simulink model "hierarchical_controll"  (R2022b)
settings: Solver=ode45  StartTime=0.0  StopTime=40  RelTol=1e-3
values from neighbouring files (symbols this model uses):
  d0 = 3.5    [planner.m]
  e_3 = [0 0 1]'    [main.m]
  g = 9.81    [main.m]
  Ib = diag([1.2416 1.2416 2*1.2416])    [main.m]
  K_attr = 0.8    [planner.m]
  K_rep = 0.6    [planner.m]
  Kp = diag([100 100 100])    [main.m]
  Kr = diag([20 20 3.5])    [main.m]
  Kv = diag([8 8 8])    [main.m]
  Kw = diag([5 6.5 2.5])    [main.m]
  lin_vel_0 = [dot_x0 dot_y0 dot_z0]    [planner.m]
  mass = 1.2    [main.m]
  obstacle_points_total = obstacle_points_total'    [planner.m]
  orient_0 = [0 0 0]    [planner.m]
  pos_0 = [x0 y0 z0]    [planner.m]
  pos_fin = [xf yf zf]    [planner.m]
  Ts = 0.001    [main.m]
  uT_0 = 11.772    [main.m]
  w_bb_0 = [0 0 0]    [planner.m]
libraries: uavsimlib x3, robotcorelib x2, uavutilslib x2, eeGeneralControl x1
settings Model: Creator=fabioruggiero  LastModifiedBy=anton
settings OptimizationCC: ReuseModelBlockBuffer=on
settings ModelReferenceCC: EnableRefExpFcnMdlSchedulingChecks=on

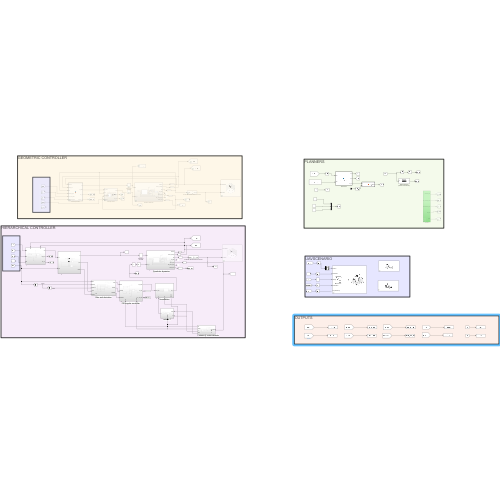
[thumbnail: Simulink's stored preview of the top-level diagram]
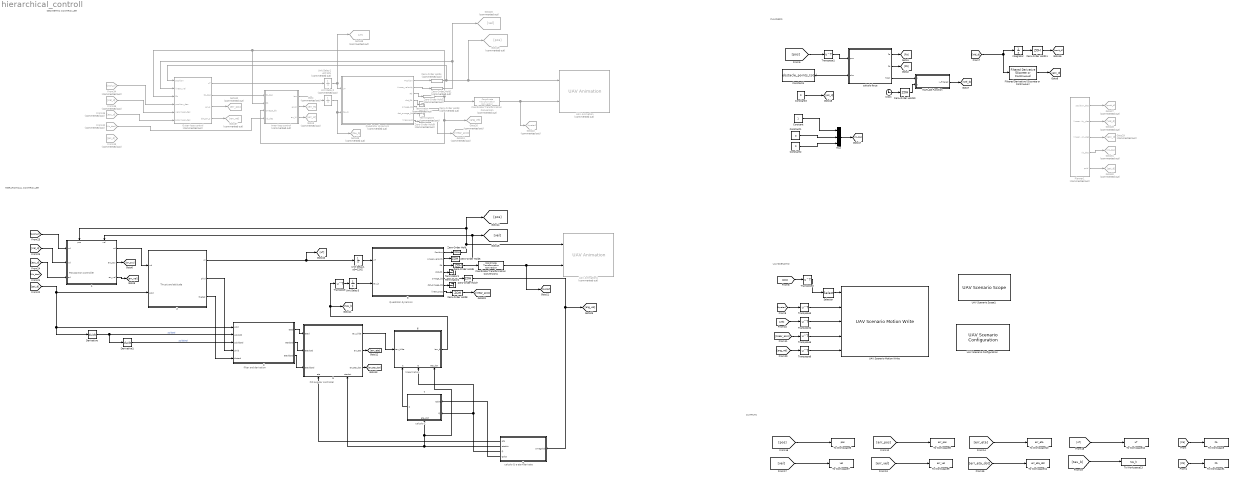
== system hierarchical_controll ==
  note: calcolo Q e eta+derivate
  note: calcolo C
  note: linearization
  note: PID angular controller
  note: Quadrotor dynamics
  note: filter and derivation
  note: Thrust and attitude
  note: PID position controller
  note: PLANNERS
  note: HIERARCHICAL CONTROLLER
  note: GEOMETRIC CONTROLLER
  note: UAVSCENARIO
  note: OUTPUTS
  "1                                                               " : Subsystem
      settings: PortSchema="{\"entries\":[{\"content\":{\"sides\":[{\"content\":{\"connectorIds\":[\"In1\",\"In2\",\"In3\"]},\"type\":\"ConnectorPlacement.EquallySpacedRectSide\",\"uuid\":\"85e0d77d-a667-4893-9520-464dcfab6198\"},{\"content\":{\"connectorIds\":[\"Out1\",\"Out2\",\"Out3\"],\"side\":\"RIGHT\"},\"type\":\"ConnectorPlacement.EquallySpacedRectSide\",\"uuid\":\"778112c6-e857-467f-a494-37829ee7f6de\"},{\"content\":{\"connectorIds\":[\"In4\",\"In5\"],\"side\":\"TOP\"},\"type\":\"ConnectorPlacement.EquallySpacedRectSide\",\"uuid\":\"7a58fbc8-384a-41ea-ad35-507457b1f60b\"}]},\"type\":\"ConnectorPlacement.EquallySpacedConnector\",\"uuid\":\"a6f9beb4-828c-454c-887a-520afea17d8a\"}],\"packageUris\":[\"http://schema.mathworks.com/mf0/Connector/R2020b\"],\"version\":\"1.0\"}"
  "2                                                       " : Subsystem
  "3                                                                                " : Subsystem
  "4                                                                          " : Subsystem
  "5                                                                   " : Subsystem
      settings: PortSchema="{\"entries\":[{\"content\":{\"sides\":[{\"content\":{\"connectorIds\":[\"In1\",\"In2\",\"In3\"]},\"type\":\"ConnectorPlacement.EquallySpacedRectSide\",\"uuid\":\"65edaed1-88f7-4380-a3c2-d91c382e58d8\"},{\"content\":{\"connectorIds\":[\"Out1\",\"Out2\",\"Out3\"],\"side\":\"RIGHT\"},\"type\":\"ConnectorPlacement.EquallySpacedRectSide\",\"uuid\":\"b4927c3a-556e-4efb-b7a2-196eb11d91c2\"},{\"content\":{\"connectorIds\":[],\"side\":\"TOP\"},\"type\":\"ConnectorPlacement.EquallySpacedRectSide\",\"uuid\":\"d0d93e72-ef33-404e-bf49-2a921e5b1f46\"},{\"content\":{\"connectorIds\":[\"In4\",\"In5\"],\"side\":\"BOTTOM\"},\"type\":\"ConnectorPlacement.EquallySpacedRectSide\",\"uuid\":\"fc2b4b79-e5bc-46f9-b483-cd3a784daa2c\"}]},\"type\":\"ConnectorPlacement.EquallySpacedConnector\",\"uuid\":\"3b418c0f-1ef1-41d2-9d0b-065cc025c1dc\"}],\"packageUris\":[\"http://schema.mathworks.com/mf0/Connector/R2020b\"],\"version\":\"1.0\"}"
  "6                                                          " : Subsystem
      settings: PortSchema="{\"entries\":[{\"content\":{\"sides\":[{\"content\":{\"connectorIds\":[\"In1\"]},\"type\":\"ConnectorPlacement.EquallySpacedRectSide\",\"uuid\":\"0beb0235-60e3-41f7-812a-43c156a669e6\"},{\"content\":{\"connectorIds\":[\"Out1\"],\"side\":\"RIGHT\"},\"type\":\"ConnectorPlacement.EquallySpacedRectSide\",\"uuid\":\"de9ad457-04ca-4167-913f-fe2cc1e03613\"},{\"content\":{\"connectorIds\":[],\"side\":\"TOP\"},\"type\":\"ConnectorPlacement.EquallySpacedRectSide\",\"uuid\":\"f1328202-7222-41d3-b6d6-2d5d11bea743\"},{\"content\":{\"connectorIds\":[\"In2\",\"In3\",\"In4\"],\"side\":\"BOTTOM\"},\"type\":\"ConnectorPlacement.EquallySpacedRectSide\",\"uuid\":\"eb41c250-0583-48fd-9f70-967dbb920771\"}]},\"type\":\"ConnectorPlacement.EquallySpacedConnector\",\"uuid\":\"65996137-7811-4a08-986c-c256136c93e4\"}],\"packageUris\":[\"http://schema.mathworks.com/mf0/Connector/R2020b\"],\"version\":\"1.0\"}"
  "7                                     " : Subsystem
      settings: PortSchema="{\"entries\":[{\"content\":{\"sides\":[{\"content\":{\"connectorIds\":[\"In1\",\"In2\"]},\"type\":\"ConnectorPlacement.EquallySpacedRectSide\",\"uuid\":\"32eaabac-cb83-4fe8-9235-f1617512dfe4\"},{\"content\":{\"connectorIds\":[\"Out1\"],\"side\":\"RIGHT\"},\"type\":\"ConnectorPlacement.EquallySpacedRectSide\",\"uuid\":\"6410da22-b624-4417-a1de-532b1b31b04c\"},{\"content\":{\"connectorIds\":[],\"side\":\"TOP\"},\"type\":\"ConnectorPlacement.EquallySpacedRectSide\",\"uuid\":\"ac47dc5b-e2fb-44dd-8524-01f66e23453c\"},{\"content\":{\"connectorIds\":[\"In3\"],\"side\":\"BOTTOM\"},\"type\":\"ConnectorPlacement.EquallySpacedRectSide\",\"uuid\":\"bde9f19c-50b2-41fa-8bff-f203ec6c7c10\"}]},\"type\":\"ConnectorPlacement.EquallySpacedConnector\",\"uuid\":\"1596106e-62b1-4910-94cd-14b1fe3e52a0\"}],\"packageUris\":[\"http://schema.mathworks.com/mf0/Connector/R2020b\"],\"version\":\"1.0\"}"
  "8                                                            " : Subsystem
  Clock : Clock
  Constant : Constant
  Constant1 : Constant  Value=0
  Constant2 : Constant  Value=0
  Constant3 : Constant  Value=0
  Constant4 : Constant  Value=obstacle_points_total
  Coordinate Transformation Conversion : robotcorelib/Coordinate Transformation Conversion  Commented=on  InputRepresentation=Rotation Matrix  InputEulerSequence=ZYX  ShowTrVecInputPort=on  OutputRepresentation=Quaternion  OutputEulerSequence=ZYX  ShowTrVecOutputPort=on  SimulateUsing=Interpreted execution
  Coordinate Transformation Conversion1 : robotcorelib/Coordinate Transformation Conversion  InputRepresentation=Rotation Matrix  InputEulerSequence=ZYX  ShowTrVecInputPort=on  OutputRepresentation=Quaternion  OutputEulerSequence=ZYX  ShowTrVecOutputPort=on  SimulateUsing=Interpreted execution
  Derivative : Derivative
  Derivative1 : Derivative
  Filtered Derivative (Discrete or Continuous) : eeGeneralControl/Filtered Derivative (Discrete or Continuous)  K=1  T=Ts  B=inf  A=-inf  minRatio=10  init_option=Specify as parameter  x0=[0,0,0]  Ts=-1
      settings: LibrarySourceBlock=|
      | ee_sl_lib/General Control/Filtered Derivative
      | (Discrete or Continuous)
  From32 : From  Commented=on  GotoTag=xb_des
  From33 : From  Commented=on  GotoTag=psi_d
  From34 : From  Commented=on  GotoTag=posit_d
  From35 : From  Commented=on  GotoTag=acc_d
  From36 : From  Commented=on  GotoTag=Vel_d
  Goto : Goto  Commented=on  GotoTag=err_R
  Goto19 : Goto  Commented=on  GotoTag=pos
  Goto20 : Goto  Commented=on  GotoTag=vel
  Goto22 : Goto  Commented=on  GotoTag=quater
  Goto24 : Goto  Commented=on  GotoTag=linear_accc
  Goto26 : Goto  Commented=on  GotoTag=ang_vel
  Goto27 : Goto  Commented=on  GotoTag=posit_d
  Goto28 : Goto  Commented=on  GotoTag=Vel_d
  Goto29 : Goto  Commented=on  GotoTag=acc_d
  Goto3 : Goto  Commented=on  GotoTag=err_W
  Goto30 : Goto  Commented=on  GotoTag=psi_d
  Goto31 : Goto  Commented=on  GotoTag=xb_des
  Goto32 : Goto  Commented=on  GotoTag=err_pos
  Goto37 : Goto  Commented=on  GotoTag=err_vel
  Goto38 : Goto  Commented=on  GotoTag=uT
  Goto39 : Goto  Commented=on  GotoTag=tau_b
  Inner-loop control : Subsystem  Commented=on
  Integrator : Integrator  InitialCondition=pos_0
  MATLAB Function : MATLAB Function  TreatAsAtomicUnit=on
  Mux : Mux  Inputs=3
  Outer-loop control : MATLAB Function  Commented=on  TreatAsAtomicUnit=on
  Planner1 : Subsystem  Commented=on
  Quadrotor dynamics : Subsystem  Commented=on
  Selector : Selector  InputPortWidth=3  IndexOptions=Index vector (dialog)  Indices=[2 1 3]  OutputSizes=1
  Terminator : Terminator  Commented=on
  Terminator1 : Terminator
  Terminator2 : Terminator
  Terminator3 : Terminator  Commented=on
  To Workspace : ToWorkspace  VariableName=Fa  SaveFormat=Timeseries  SampleTime=-1
  To Workspace1 : ToWorkspace  VariableName=Fb  SaveFormat=Timeseries  SampleTime=-1
  To Workspace10 : ToWorkspace  VariableName=err_eta  SaveFormat=Timeseries  SampleTime=-1
  To Workspace11 : ToWorkspace  VariableName=err_eta_dot  SaveFormat=Timeseries  SampleTime=-1
  To Workspace12 : ToWorkspace  VariableName=uT  SaveFormat=Timeseries  SampleTime=-1
  To Workspace13 : ToWorkspace  VariableName=tau_b  SaveFormat=Timeseries  SampleTime=-1
  To Workspace6 : ToWorkspace  VariableName=pos  SaveFormat=Timeseries  SampleTime=-1
  To Workspace7 : ToWorkspace  VariableName=vel  SaveFormat=Timeseries  SampleTime=-1
  To Workspace8 : ToWorkspace  VariableName=err_pos  SaveFormat=Timeseries  SampleTime=-1
  To Workspace9 : ToWorkspace  VariableName=err_vel  SaveFormat=Timeseries  SampleTime=-1
  Transpose{,1..6} (7 alike) : Math  Operator=transpose
  UAV Animation : uavutilslib/UAV Animation  Commented=on  UAVType=Multirotor  UAVSize=1  InertialZDirection=Down  SampleTime=0.1
  UAV Animation1 : uavutilslib/UAV Animation  Commented=on  UAVType=Multirotor  UAVSize=2  InertialZDirection=Down  SampleTime=0.1
  UAV Scenario Configuration : uavsimlib/UAV Scenario Configuration  Priority=-1  UAVScenarioObject=piazza  SampleTime=Ts  UpdateParam=false  SensorMotionBusName='SensorMotionBus'  PlatformMotionBusName='PlatformMotionBus'  ScenarioMotionBusName='ScenarioMotionBus'  ScenarioMotionSignalName='ScenarioMotions'
  UAV Scenario Motion Write : uavsimlib/UAV Scenario Motion Write  Priority=0  PlatName='UAV_platform'  ReferenceFrame=NED
  UAV Scenario Scope1 : uavsimlib/UAV Scenario Scope  Priority=1  SensorNameTable={}  SampleTime=0.1
  Unit Delay1 u0=12N : UnitDelay  Commented=on  InitialCondition=uT_0  SampleTime=Ts
  Unit Delay1 u0=12N2 : UnitDelay  InitialCondition=uT_0  SampleTime=Ts
  Unit Delay2 : UnitDelay  Commented=on  InitialCondition=[0 0 0]  SampleTime=Ts
  Unit Delay3 : UnitDelay  InitialCondition=[0 0 0]  SampleTime=Ts
  Zero-Order Hold{,5..8,10..11} (7 alike) : ZeroOrderHold  SampleTime=Ts
  Zero-Order Hold{1..4,9} (5 alike) : ZeroOrderHold  Commented=on  SampleTime=Ts
  calcolo forza : MATLAB Function  TreatAsAtomicUnit=on
  wires:
  Outer-loop control/1(uT) -> Unit Delay1 u0=12N/1
  Unit Delay1 u0=12N/1 -> Goto38/1, Quadrotor dynamics/1(uT)
  Quadrotor dynamics/1(Position) -> Zero-Order Hold4/1
  Quadrotor dynamics/2(Linear_velocity) -> Zero-Order Hold1/1
  Quadrotor dynamics/5(omega_bb) -> Zero-Order Hold3/1
  Zero-Order Hold4/1 -> Goto19/1, UAV Animation/1, Outer-loop control/1(position)
  Zero-Order Hold1/1 -> Goto20/1, Outer-loop control/2(linear_vel)
  Quadrotor dynamics/3(Rb) -> Zero-Order Hold2/1
  Unit Delay2/1 -> Goto39/1, Quadrotor dynamics/2(tau_b)
  Quadrotor dynamics/4(dot_Rb) -> Terminator/1
  Outer-loop control/3(err_p) -> Goto32/1
  Outer-loop control/4(dot_err_p) -> Goto37/1
  Quadrotor dynamics/6(dot_omega_bb) -> Terminator3/1
  Coordinate Transformation Conversion/1 -> Goto22/1, UAV Animation/2
  Outer-loop control/2(zb_des) -> Inner-loop control/1(zb_des)
  Zero-Order Hold3/1 -> Inner-loop control/3(omega_bb), Goto26/1
  Inner-loop control/1(tau) -> Unit Delay2/1
  Inner-loop control/2(err_R) -> Goto/1
  Inner-loop control/3(err_W) -> Goto3/1
  Coordinate Transformation Conversion1/1 -> [quater], UAV Animation1/2
  "3                                                                                "/6(dot_omega_bb) -> Terminator2/1
  "3                                                                                "/4(dot_Rb) -> Terminator1/1
  "6                                                          "/1(tau_b) -> Transpose/1, [tau_b]
  Zero-Order Hold/1 -> [pos], "1                                                               "/4(pos), UAV Animation1/1
  "3                                                                                "/5(omega_bb) -> Zero-Order Hold7/1
  "3                                                                                "/3(Rb) -> Zero-Order Hold6/1
  "3                                                                                "/2(Linear_velocity) -> Zero-Order Hold5/1
  "3                                                                                "/1(Position) -> Zero-Order Hold/1
  "2                                                       "/1(ut) -> [uT], Unit Delay1 u0=12N2/1
  Zero-Order Hold5/1 -> "1                                                               "/5(vel), [vel]
  "1                                                               "/1(ud) -> "2                                                       "/1(ud)
  Derivative/1 -> Derivative1/1, "4                                                                          "/2(psidotd)  "psidotd"
  Derivative1/1 -> "4                                                                          "/3(psiddotd)  "psiddotd"
  "2                                                       "/3(thetad) -> "4                                                                          "/5(thetad)
  "2                                                       "/2(phid) -> "4                                                                          "/4(phid)
  "4                                                                          "/1(etad) -> "5                                                                   "/1(etad)
  "4                                                                          "/2(etadotd) -> "5                                                                   "/2(etadotd)
  "4                                                                          "/3(etaddotd) -> "5                                                                   "/3(etaddotd)
  "8                                                            "/1(eta) -> "5                                                                   "/4(eta)
  "8                                                            "/2(etadot) -> "5                                                                   "/5(etadot), "6                                                          "/4(eta_dot), "7                                     "/3(eta_dot)
  "5                                                                   "/1(tau_tilde) -> "6                                                          "/1(tau_tilde)
  "8                                                            "/3(Q) -> "6                                                          "/3(Q), "7                                     "/2(Q)
  "8                                                            "/4(Qdot) -> "7                                     "/1(Qdot)
  "7                                     "/1(C) -> "6                                                          "/2(C)
  Zero-Order Hold7/1 -> "8                                                            "/1(omegabb), [ang_vel]
  Unit Delay3/1 -> "3                                                                                "/2(tau_b)
  Unit Delay1 u0=12N2/1 -> "3                                                                                "/1(uT)
  [pos] -> To Workspace6/1
  [vel] -> To Workspace7/1
  [err_pos] -> To Workspace8/1
  [err_vel] -> To Workspace9/1
  [err_eta] -> To Workspace10/1
  [err_eta_dot] -> To Workspace11/1
  [uT] -> To Workspace12/1
  [tau_b] -> To Workspace13/1
  "1                                                               "/2(err_pos) -> [err_pos]
  "1                                                               "/3(err_vel) -> [err_vel]
  "5                                                                   "/2(err_eta) -> [err_eta]
  "5                                                                   "/3(err_eta_dot) -> [err_eta_dot]
  Transpose/1 -> Unit Delay3/1
  Constant4/1 -> calcolo forza/2(obs)
  [pos] -> Transpose1/1
  Transpose1/1 -> calcolo forza/1(pos)
  calcolo forza/1(Fa) -> [Fa]
  calcolo forza/2(Fb) -> [Fb]
  [Vel_d] -> Integrator/1, Filtered Derivative (Discrete or Continuous)/1
  Filtered Derivative (Discrete or Continuous)/1 -> [acc_d]
  Constant1/1 -> Mux/2
  Constant2/1 -> Mux/3
  Constant/1 -> Mux/1
  Mux/1 -> [xb_des]
  Constant3/1 -> [psi_d]
  Transpose2/1 -> Selector/1
  [pos] -> Transpose2/1
  [quater] -> Transpose3/1
  [vel] -> Transpose4/1
  Transpose4/1 -> UAV Scenario Motion Write/3
  "3                                                                                "/7(linear_accc) -> Zero-Order Hold8/1
  Quadrotor dynamics/7(linear_acc) -> Zero-Order Hold9/1
  [linear_accc] -> Transpose5/1
  Transpose5/1 -> UAV Scenario Motion Write/4
  [ang_vel] -> Transpose6/1
  Transpose6/1 -> UAV Scenario Motion Write/5
  Zero-Order Hold6/1 -> Coordinate Transformation Conversion1/1
  Transpose3/1 -> UAV Scenario Motion Write/2
  [posit_d] -> "1                                                               "/1(xd)
  [acc_d] -> "1                                                               "/3(ad)
  [Vel_d] -> "1                                                               "/2(vd)
  [psi_d] -> "2                                                       "/2(psid), "4                                                                          "/1(psid), Derivative/1
  Zero-Order Hold8/1 -> [linear_accc]
  From34/1 -> Outer-loop control/4(position_des)
  From36/1 -> Outer-loop control/5(vel_linear_des)
  From35/1 -> Outer-loop control/6(acc_linear_des)
  From32/1 -> Inner-loop control/4(xb_des)
  Zero-Order Hold9/1 -> Goto24/1
  Zero-Order Hold2/1 -> Coordinate Transformation Conversion/1, Inner-loop control/2(Rb), Outer-loop control/3(Rb)
  Clock/1 -> Zero-Order Hold10/1
  calcolo forza/3(F_tot) -> MATLAB Function/1(x)
  MATLAB Function/1(x_filtered) -> [Vel_d]
  Zero-Order Hold10/1 -> MATLAB Function/2(t)
  Zero-Order Hold11/1 -> [posit_d]
  Integrator/1 -> Zero-Order Hold11/1
  Planner1/5(psid) -> Goto30/1
  Planner1/4(xb_des) -> Goto31/1
  Planner1/3(linear_acceleration_des) -> Goto29/1
  Planner1/2(linear_velocity_des) -> Goto28/1
  Planner1/1(position_des) -> Goto27/1
  Selector/1 -> UAV Scenario Motion Write/1
  [Fa] -> To Workspace/1
  [Fb] -> To Workspace1/1

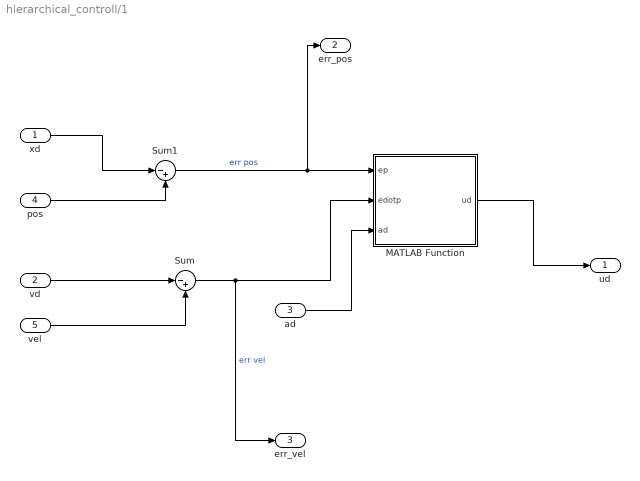
== system hierarchical_controll/1                                                                ==
  xd : Inport
  vd : Inport  Port=2
  ad : Inport  Port=3
  pos : Inport  Port=4
  vel : Inport  Port=5
  MATLAB Function : MATLAB Function  TreatAsAtomicUnit=on
  Sum : Sum  Inputs=|-+
  Sum1 : Sum  Inputs=|-+
  ud : Outport
  err_pos : Outport  Port=2
  err_vel : Outport  Port=3
  wires:
  vd/1 -> Sum/1
  vel/1 -> Sum/2
  xd/1 -> Sum1/1
  pos/1 -> Sum1/2
  Sum1/1 -> err_pos/1, MATLAB Function/1(ep)  "err pos"
  Sum/1 -> err_vel/1, MATLAB Function/2(edotp)  "err vel"
  ad/1 -> MATLAB Function/3(ad)
  MATLAB Function/1(ud) -> ud/1

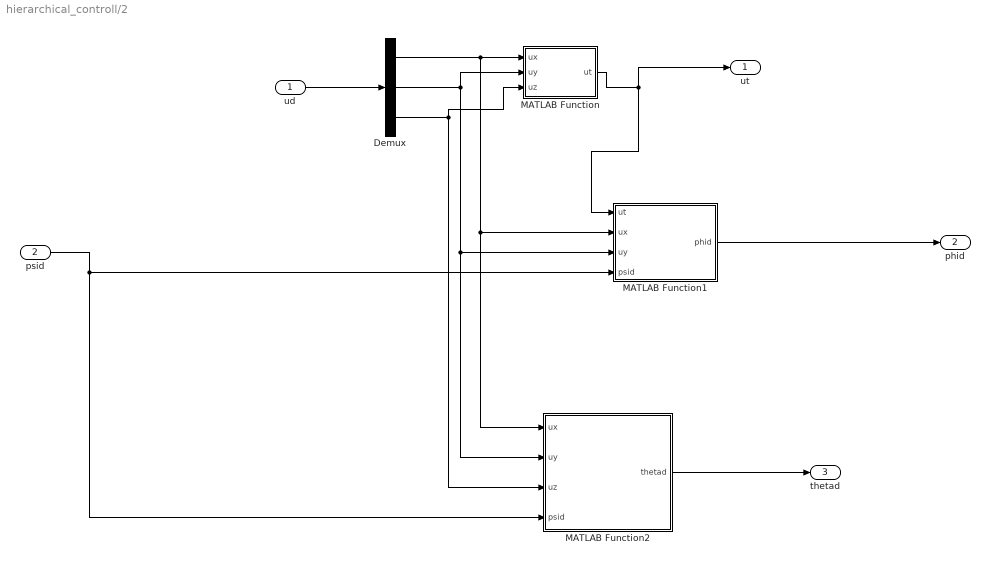
== system hierarchical_controll/2                                                        ==
  ud : Inport
  psid : Inport  Port=2
  Demux : Demux  Outputs=3
  MATLAB Function : MATLAB Function  TreatAsAtomicUnit=on
  MATLAB Function1 : MATLAB Function  TreatAsAtomicUnit=on
  MATLAB Function2 : MATLAB Function  TreatAsAtomicUnit=on
  ut : Outport
  phid : Outport  Port=2
  thetad : Outport  Port=3
  wires:
  ud/1 -> Demux/1
  Demux/1 -> MATLAB Function2/1(ux), MATLAB Function1/2(ux), MATLAB Function/1(ux)
  Demux/2 -> MATLAB Function2/2(uy), MATLAB Function1/3(uy), MATLAB Function/2(uy)
  Demux/3 -> MATLAB Function2/3(uz), MATLAB Function/3(uz)
  MATLAB Function/1(ut) -> MATLAB Function1/1(ut), ut/1
  psid/1 -> MATLAB Function2/4(psid), MATLAB Function1/4(psid)
  MATLAB Function2/1(thetad) -> thetad/1
  MATLAB Function1/1(phid) -> phid/1

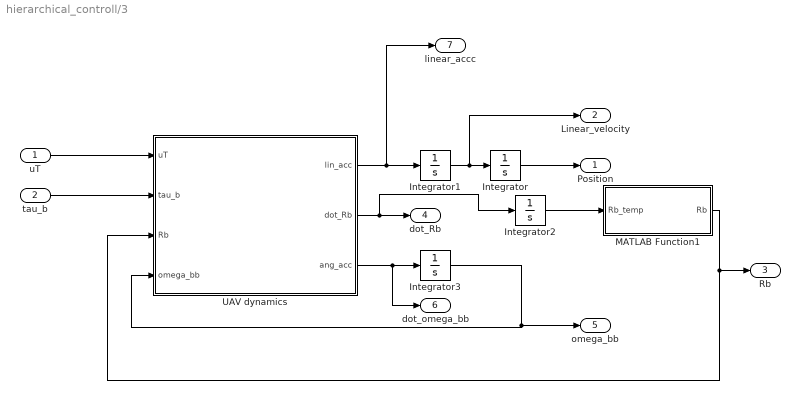
== system hierarchical_controll/3                                                                                 ==
  uT : Inport
  tau_b : Inport  Port=2
  Integrator : Integrator  InitialCondition=pos_0
  Integrator1 : Integrator  InitialCondition=lin_vel_0
  Integrator2 : Integrator  InitialCondition=eul2rotm(orient_0)
  Integrator3 : Integrator  InitialCondition=w_bb_0
  MATLAB Function1 : MATLAB Function  TreatAsAtomicUnit=on
  UAV dynamics : MATLAB Function  TreatAsAtomicUnit=on
  Position : Outport
  Linear_velocity : Outport  Port=2
  Rb : Outport  Port=3
  dot_Rb : Outport  Port=4
  omega_bb : Outport  Port=5
  dot_omega_bb : Outport  Port=6
  linear_accc : Outport  Port=7
  wires:
  Integrator2/1 -> MATLAB Function1/1(Rb_temp)
  MATLAB Function1/1(Rb) -> UAV dynamics/3(Rb), Rb/1
  UAV dynamics/2(dot_Rb) -> dot_Rb/1, Integrator2/1
  Integrator3/1 -> omega_bb/1, UAV dynamics/4(omega_bb)
  Integrator1/1 -> Integrator/1, Linear_velocity/1
  uT/1 -> UAV dynamics/1(uT)
  UAV dynamics/1(lin_acc) -> linear_accc/1, Integrator1/1
  UAV dynamics/3(ang_acc) -> Integrator3/1, dot_omega_bb/1
  Integrator/1 -> Position/1
  tau_b/1 -> UAV dynamics/2(tau_b)

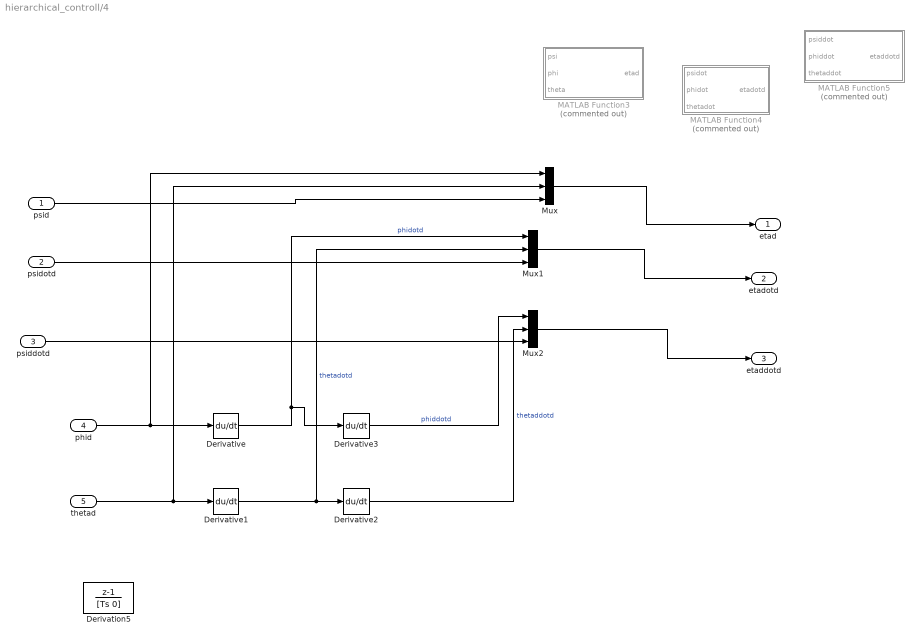
== system hierarchical_controll/4                                                                           ==
  psid : Inport
  psidotd : Inport  Port=2
  psiddotd : Inport  Port=3
  phid : Inport  Port=4
  thetad : Inport  Port=5
  Derivation5 : DiscreteTransferFcn  Numerator=[1 -1]  Denominator=[Ts 0]  SampleTime=Ts
  Derivative{,1..3} (4 alike) : Derivative
  MATLAB Function3 : MATLAB Function  Commented=on  TreatAsAtomicUnit=on
  MATLAB Function4 : MATLAB Function  Commented=on  TreatAsAtomicUnit=on
  MATLAB Function5 : MATLAB Function  Commented=on  TreatAsAtomicUnit=on
  Mux : Mux  Inputs=3
  Mux1 : Mux  Inputs=3
  Mux2 : Mux  Inputs=3
  etad : Outport
  etadotd : Outport  Port=2
  etaddotd : Outport  Port=3
  wires:
  phid/1 -> Mux/1, Derivative/1
  thetad/1 -> Mux/2, Derivative1/1
  Derivative1/1 -> Mux1/2, Derivative2/1  "thetadotd"
  Derivative/1 -> Mux1/1, Derivative3/1  "phidotd"
  Derivative3/1 -> Mux2/1  "phiddotd"
  Derivative2/1 -> Mux2/2  "thetaddotd"
  psidotd/1 -> Mux1/3
  psiddotd/1 -> Mux2/3
  Mux/1 -> etad/1
  Mux2/1 -> etaddotd/1
  psid/1 -> Mux/3
  Mux1/1 -> etadotd/1

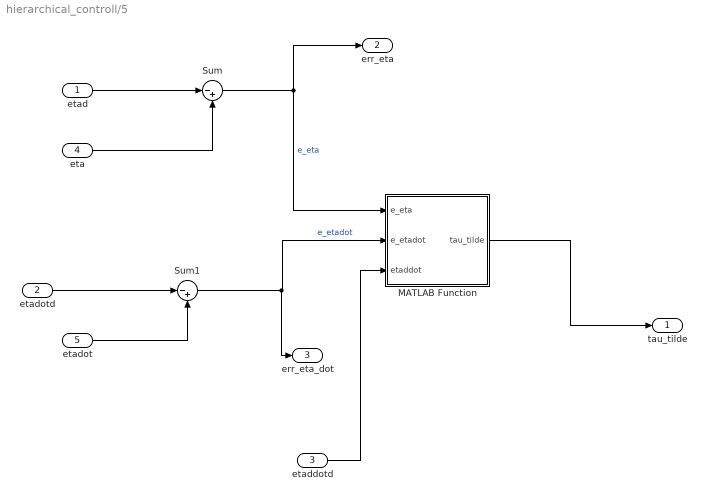
== system hierarchical_controll/5                                                                    ==
  etad : Inport
  etadotd : Inport  Port=2
  etaddotd : Inport  Port=3
  eta : Inport  Port=4
  etadot : Inport  Port=5
  MATLAB Function : MATLAB Function  TreatAsAtomicUnit=on
  Sum : Sum  Inputs=|-+
  Sum1 : Sum  Inputs=|-+
  tau_tilde : Outport
  err_eta : Outport  Port=2
  err_eta_dot : Outport  Port=3
  wires:
  etad/1 -> Sum/1
  eta/1 -> Sum/2
  etadotd/1 -> Sum1/1
  Sum/1 -> MATLAB Function/1(e_eta), err_eta/1  "e_eta"
  Sum1/1 -> err_eta_dot/1, MATLAB Function/2(e_etadot)  "e_etadot"
  MATLAB Function/1(tau_tilde) -> tau_tilde/1
  etadot/1 -> Sum1/2
  etaddotd/1 -> MATLAB Function/3(etaddot)

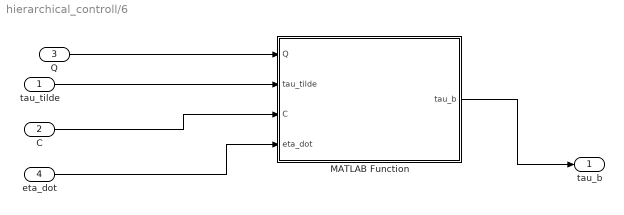
== system hierarchical_controll/6                                                           ==
  tau_tilde : Inport
  C : Inport  Port=2
  Q : Inport  Port=3
  eta_dot : Inport  Port=4
  MATLAB Function : MATLAB Function  TreatAsAtomicUnit=on
  tau_b : Outport
  wires:
  eta_dot/1 -> MATLAB Function/4(eta_dot)
  C/1 -> MATLAB Function/3(C)
  tau_tilde/1 -> MATLAB Function/2(tau_tilde)
  Q/1 -> MATLAB Function/1(Q)
  MATLAB Function/1(tau_b) -> tau_b/1

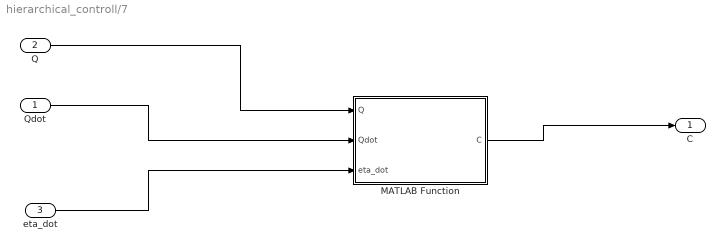
== system hierarchical_controll/7                                      ==
  Qdot : Inport
  Q : Inport  Port=2
  eta_dot : Inport  Port=3
  MATLAB Function : MATLAB Function  TreatAsAtomicUnit=on
  C : Outport
  wires:
  MATLAB Function/1(C) -> C/1
  Q/1 -> MATLAB Function/1(Q)
  Qdot/1 -> MATLAB Function/2(Qdot)
  eta_dot/1 -> MATLAB Function/3(eta_dot)

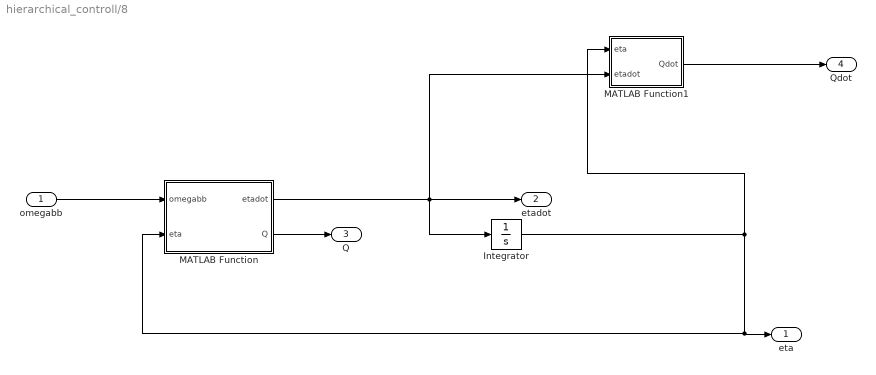
== system hierarchical_controll/8                                                             ==
  omegabb : Inport
  Integrator : Integrator  InitialCondition=[0, 0, 0]'
  MATLAB Function : MATLAB Function  TreatAsAtomicUnit=on
  MATLAB Function1 : MATLAB Function  TreatAsAtomicUnit=on
  eta : Outport
  etadot : Outport  Port=2
  Q : Outport  Port=3
  Qdot : Outport  Port=4
  wires:
  omegabb/1 -> MATLAB Function/1(omegabb)
  MATLAB Function/1(etadot) -> MATLAB Function1/2(etadot), Integrator/1, etadot/1
  MATLAB Function/2(Q) -> Q/1
  MATLAB Function1/1(Qdot) -> Qdot/1
  Integrator/1 -> MATLAB Function/2(eta), eta/1, MATLAB Function1/1(eta)

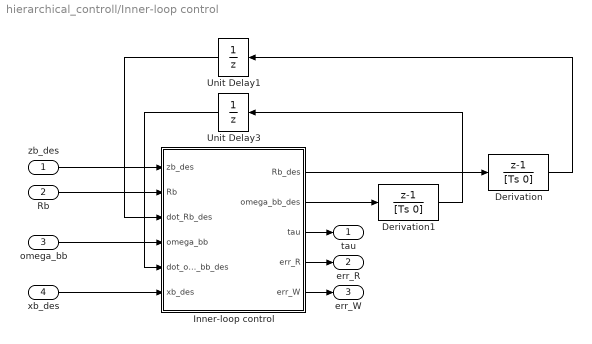
== system hierarchical_controll/Inner-loop control ==
  zb_des : Inport
  Rb : Inport  Port=2
  omega_bb : Inport  Port=3
  xb_des : Inport  Port=4
  Derivation : DiscreteTransferFcn  Numerator=[1 -1]  Denominator=[Ts 0]  InitialStates=[1 0 0;0 1 0;0 0 1]  SampleTime=Ts
  Derivation1 : DiscreteTransferFcn  Numerator=[1 -1]  Denominator=[Ts 0]  InitialStates=[0 0 0]  SampleTime=Ts
  Inner-loop control : MATLAB Function  TreatAsAtomicUnit=on
  Unit Delay1 : UnitDelay  InitialCondition=eye(3)  SampleTime=Ts
  Unit Delay3 : UnitDelay  InitialCondition=[0 0 0]  SampleTime=Ts
  tau : Outport
  err_R : Outport  Port=2
  err_W : Outport  Port=3
  wires:
  xb_des/1 -> Inner-loop control/6(xb_des)
  Inner-loop control/4(err_R) -> err_R/1
  Rb/1 -> Inner-loop control/2(Rb)
  Inner-loop control/3(tau) -> tau/1
  Unit Delay1/1 -> Inner-loop control/3(dot_Rb_des)
  Derivation1/1 -> Unit Delay3/1
  Inner-loop control/5(err_W) -> err_W/1
  Unit Delay3/1 -> Inner-loop control/5(dot_omega_bb_des)
  Derivation/1 -> Unit Delay1/1
  zb_des/1 -> Inner-loop control/1(zb_des)
  omega_bb/1 -> Inner-loop control/4(omega_bb)
  Inner-loop control/1(Rb_des) -> Derivation/1
  Inner-loop control/2(omega_bb_des) -> Derivation1/1

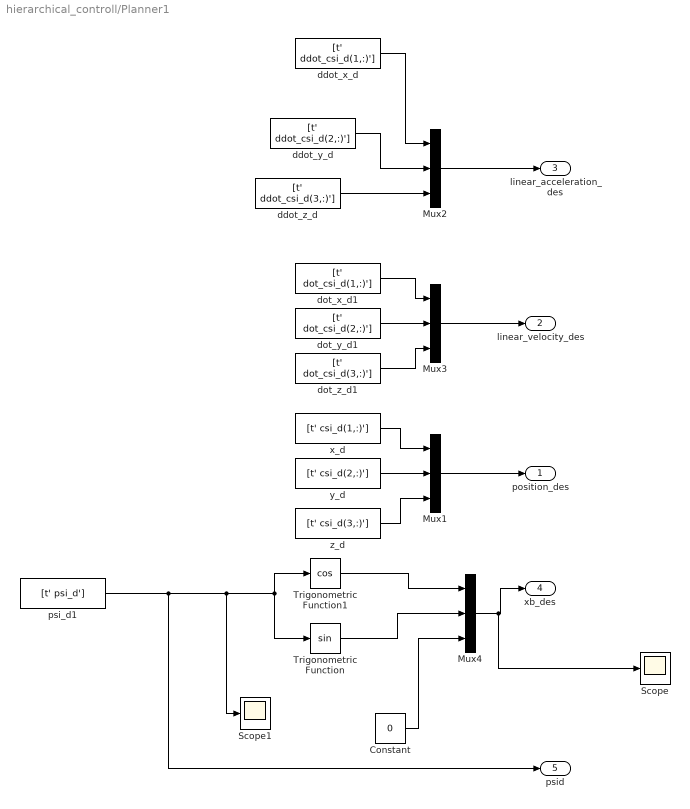
== system hierarchical_controll/Planner1 ==
  Constant : Constant  Value=0
  Mux{1..4} (4 alike) : Mux  Inputs=3
  Scope : Scope
  Scope1 : Scope
  Trigonometric Function : Trigonometry
  Trigonometric Function1 : Trigonometry  Operator=cos
  ddot_x_d : FromWorkspace  VariableName=[t' ddot_csi_d(1,:)']  SampleTime=Ts
  ddot_y_d : FromWorkspace  VariableName=[t' ddot_csi_d(2,:)']  SampleTime=Ts
  ddot_z_d : FromWorkspace  VariableName=[t' ddot_csi_d(3,:)']  SampleTime=Ts
  dot_x_d1 : FromWorkspace  VariableName=[t' dot_csi_d(1,:)']  SampleTime=Ts
  dot_y_d1 : FromWorkspace  VariableName=[t' dot_csi_d(2,:)']  SampleTime=Ts
  dot_z_d1 : FromWorkspace  VariableName=[t' dot_csi_d(3,:)']  SampleTime=Ts
  psi_d1 : FromWorkspace  VariableName=[t' psi_d']  SampleTime=Ts
  x_d : FromWorkspace  VariableName=[t' csi_d(1,:)']  SampleTime=Ts
  y_d : FromWorkspace  VariableName=[t' csi_d(2,:)']  SampleTime=Ts
  z_d : FromWorkspace  VariableName=[t' csi_d(3,:)']  SampleTime=Ts
  position_des : Outport
  linear_velocity_des : Outport  Port=2
  linear_acceleration_des : Outport  Port=3
  xb_des : Outport  Port=4
  psid : Outport  Port=5
  wires:
  Constant/1 -> Mux4/3
  Trigonometric Function1/1 -> Mux4/1
  psi_d1/1 -> psid/1, Scope1/1, Trigonometric Function/1, Trigonometric Function1/1
  Trigonometric Function/1 -> Mux4/2
  Mux4/1 -> Scope/1, xb_des/1
  Mux3/1 -> linear_velocity_des/1
  dot_x_d1/1 -> Mux3/1
  dot_z_d1/1 -> Mux3/3
  dot_y_d1/1 -> Mux3/2
  Mux1/1 -> position_des/1
  Mux2/1 -> linear_acceleration_des/1
  ddot_x_d/1 -> Mux2/1
  ddot_z_d/1 -> Mux2/3
  ddot_y_d/1 -> Mux2/2
  x_d/1 -> Mux1/1
  z_d/1 -> Mux1/3
  y_d/1 -> Mux1/2

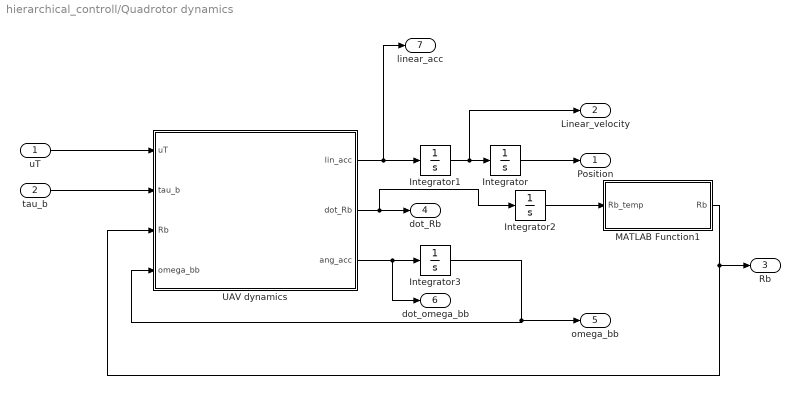
== system hierarchical_controll/Quadrotor dynamics ==
  uT : Inport
  tau_b : Inport  Port=2
  Integrator : Integrator  InitialCondition=pos_0
  Integrator1 : Integrator  InitialCondition=lin_vel_0
  Integrator2 : Integrator  InitialCondition=eul2rotm(orient_0)
  Integrator3 : Integrator  InitialCondition=w_bb_0
  MATLAB Function1 : MATLAB Function  TreatAsAtomicUnit=on
  UAV dynamics : MATLAB Function  TreatAsAtomicUnit=on
  Position : Outport
  Linear_velocity : Outport  Port=2
  Rb : Outport  Port=3
  dot_Rb : Outport  Port=4
  omega_bb : Outport  Port=5
  dot_omega_bb : Outport  Port=6
  linear_acc : Outport  Port=7
  wires:
  tau_b/1 -> UAV dynamics/2(tau_b)
  Integrator/1 -> Position/1
  UAV dynamics/3(ang_acc) -> dot_omega_bb/1, Integrator3/1
  UAV dynamics/1(lin_acc) -> linear_acc/1, Integrator1/1
  uT/1 -> UAV dynamics/1(uT)
  Integrator1/1 -> Linear_velocity/1, Integrator/1
  Integrator3/1 -> UAV dynamics/4(omega_bb), omega_bb/1
  UAV dynamics/2(dot_Rb) -> Integrator2/1, dot_Rb/1
  MATLAB Function1/1(Rb) -> Rb/1, UAV dynamics/3(Rb)
  Integrator2/1 -> MATLAB Function1/1(Rb_temp)

== matlab function hierarchical_controll/3                                                                                /MATLAB Function1 ==
  data: Rb_temp input; Rb output
function Rb = fcn(Rb_temp)
    [U,S,V] = svd(Rb_temp);
    sigma = det(U*V');
    S_ = diag([1 1 sigma]);

    Rb = U*S_*V';
end

== matlab function hierarchical_controll/3                                                                                /UAV dynamics ==
  data: uT input size=1; tau_b input size=3; lin_acc output size=3; Rb input size=[3,3]; omega_bb input size=3; dot_Rb output size=[3,3]; ang_acc output size=3; mass parameter size=1; Ib parameter size=[3,3]
function [lin_acc, dot_Rb, ang_acc] = fcn(uT,tau_b,Rb,omega_bb,mass, Ib)

lin_acc = 9.81*[0 0 1]'-(uT/mass)*Rb*[0 0 1]';
dot_Rb = Rb*skew(omega_bb);
ang_acc = inv(Ib)*(-skew(omega_bb)*Ib*omega_bb + tau_b);

end

function S = skew(v)
if(numel(v)~= 1)
S= [0 -v(3) v(2); 
    v(3) 0 -v(1);
    -v(2) v(1) 0];
else
S= zeros(3);
end
end

== matlab function hierarchical_controll/2                                                       /MATLAB Function ==
  data: ux input; ut output; uy input; uz input; mass parameter; g parameter
function ut = Calcolo_ut(ux,uy,uz, mass, g)

ut = mass*sqrt((ux^2)+(uy^2)+((uz-g)^2));

== matlab function hierarchical_controll/2                                                       /MATLAB Function1 ==
  data: ut input; phid output; ux input; uy input; psid input; mass parameter
function phid = Calcolo_phi(ut,ux,uy,psid, mass)


phid = asin((mass/ut)*(uy*cos(psid)-ux*sin(psid)));

== matlab function hierarchical_controll/2                                                       /MATLAB Function2 ==
  data: ux input; thetad output; uy input; uz input; psid input; g parameter
function thetad = Calcolo_theta(ux,uy,uz,psid, g)

thetad = atan((ux*cos(psid)+uy*sin(psid))/(uz-g));

== matlab function hierarchical_controll/calcolo forza ==
  data: pos input; Fa output; obs input; Fb output; F_tot output; K_attr parameter; K_rep parameter; pos_fin parameter; d0 parameter
function [Fa, Fb, F_tot] = calculate_force(pos, obs, K_attr, K_rep, pos_fin, d0)

errpos = pos_fin-pos;

if(norm(errpos)<1)
    Fa=K_attr*errpos;
else
    Fa=K_attr*errpos/norm(errpos);
end

gamma=3;


    Fb=zeros(1,3);


for i=1:size(obs,1)
    
    temp_obs=obs(i,:);

    distance=norm(pos-temp_obs);

    if (distance<d0)
        temp_eta=distance;
        grad=(pos-temp_obs)/distance;

        Fb=Fb+(K_rep/(temp_eta^2))*(1/temp_eta-1/d0)^(gamma-1)*grad;   
    end
end

F_tot=Fa+Fb;

end

== matlab function hierarchical_controll/MATLAB Function ==
  data: x input; x_filtered output; t input

function x_filtered = e_mov_average_filter(x, t)
    
    t_max=40;
    alpha_min=0.000001;
    alpha_max=0.07;
    
    
    
    % Calcola il valore di alpha al tempo t
    alpha = alpha_min + (alpha_max - alpha_min) * (t / t_max);

    % Inizializza la variabile persistente
    persistent x_filtered_prev
    
    % Se è la prima chiamata, inizializza la variabile persistente
    if isempty(x_filtered_prev)
        x_filtered_prev = [0 0 0];
    end
    
    % Applica il filtro a media mobile esponenziale elemento per elemento
    x_filtered = (1 - alpha) * x_filtered_prev + alpha * x;
    
    % Aggiorna la variabile persistente
    x_filtered_prev = x_filtered;
end

== matlab function hierarchical_controll/8                                                            /MATLAB Function1 ==
  data: eta input; Qdot output; etadot input
function Qdot = fcn(eta, etadot)

Qdot=[0, 0, -cos(eta(2))*etadot(2);
       0, -sin(eta(1))*etadot(1), -sin(eta(2))*sin(eta(1))*etadot(2)+cos(eta(2))*cos(eta(1))*etadot(1);
       0, -cos(eta(1))*etadot(1), -sin(eta(2))*cos(eta(1))*etadot(2)-cos(eta(2))*sin(eta(1))*etadot(1)];

== matlab function hierarchical_controll/4                                                                          /MATLAB Function3 ==
  data: psi input; etad output; phi input; theta input
function etad = fcn(psi, phi, theta)

etad = [phi; theta; psi] ;

== matlab function hierarchical_controll/5                                                                   /MATLAB Function ==
  data: e_eta input; tau_tilde output; e_etadot input; etaddot input; newKE parameter
function tau_tilde = fcn(e_eta,e_etadot,etaddot, newKE)

new_eta=[e_eta; e_etadot];


tau_tilde = -newKE*new_eta+etaddot;

== matlab function hierarchical_controll/4                                                                          /MATLAB Function4 ==
  data: psidot input; etadotd output; phidot input; thetadot input
function etadotd = fcn(psidot, phidot, thetadot)

etadotd = [phidot; thetadot; psidot] ;

== matlab function hierarchical_controll/7                                     /MATLAB Function ==
  data: Q input; C output; Qdot input; eta_dot input; Ib parameter
function C = fcn(Q, Qdot, eta_dot, Ib)

   S = skew(Q*eta_dot);
    C = Q'*S*Ib*Q + Q'*Ib*Qdot; 
    
end



function S = skew(v)
if(numel(v)~= 1)
S= [0 -v(3) v(2); 
    v(3) 0 -v(1);
    -v(2) v(1) 0];
else
S= zeros(3);
end
end

== matlab function hierarchical_controll/6                                                          /MATLAB Function ==
  data: Q input; tau_b output; tau_tilde input; C input; eta_dot input; Ib parameter
function tau_b = calcolo_tau_b(Q, tau_tilde, C, eta_dot, Ib)

tau_b = Ib*Q*tau_tilde+(inv(Q))'*C*eta_dot;

== matlab function hierarchical_controll/4                                                                          /MATLAB Function5 ==
  data: psiddot input; etaddotd output; phiddot input; thetaddot input
function etaddotd = fcn(psiddot, phiddot, thetaddot)

etaddotd = [phiddot; thetaddot; psiddot] ;

== matlab function hierarchical_controll/8                                                            /MATLAB Function ==
  data: omegabb input; etadot output; eta input; Q output
function [etadot, Q]   = fcn(omegabb, eta)

% phi= eta(1,1);
% theta= eta(2,1);
% psi=eta(3,1);



    Q=[1,              0,               -sin(eta(2));
       0,  cos(eta(1)),  cos(eta(2))*sin(eta(1));
       0, -sin(eta(1)),  cos(eta(1))*cos(eta(2))];





etadot=inv(Q)*omegabb;

== matlab function hierarchical_controll/Quadrotor dynamics/UAV dynamics ==
  data: uT input size=1; tau_b input size=3; lin_acc output size=3; Rb input size=[3,3]; omega_bb input size=3; dot_Rb output size=[3,3]; ang_acc output size=3; mass parameter size=1; Ib parameter size=[3,3]
function [lin_acc, dot_Rb, ang_acc] = fcn(uT,tau_b,Rb,omega_bb,mass, Ib)

lin_acc = 9.81*[0 0 1]'-(uT/mass)*Rb*[0 0 1]';
dot_Rb = Rb*skew(omega_bb);
ang_acc = inv(Ib)*(-skew(omega_bb)*Ib*omega_bb + tau_b);

end

function S = skew(v)
if(numel(v)~= 1)
S= [0 -v(3) v(2); 
    v(3) 0 -v(1);
    -v(2) v(1) 0];
else
S= zeros(3);
end
end

== matlab function hierarchical_controll/Outer-loop control ==
  data: position input size=3; uT output size=1; linear_vel input size=3; Rb input size=[3,3]; zb_des output size=3; mass parameter size=1; position_des input size=3; vel_linear_des input size=3; acc_linear_des input size=3; err_p output size=3; dot_err_p output size=3; Kp parameter; Kv parameter; g parameter; e_3 parameter
function [uT, zb_des, err_p, dot_err_p] = fcn(position, linear_vel, Rb, mass, ...
    position_des, vel_linear_des, acc_linear_des, Kp, Kv, g, e_3)

%% WRITE HERE THE OUTER-LOOP CONTROL
% position: linear position measure
% linear_vel: linear velocity measure
% Rb: current rotation matrix
% mass: mass of the UAV
% positon_des: desired linear position from the planner
% vel_linear_des: desired linear velocity from the planner
% acc_linear_des: desired linear acceleration from the planner
% ---
% uT: commanded total thrust
% zb_des: desired z-axis of the body frame
% err_p: position error
% dot_err_p: time derivative of the positon error

%% outer loop

err_p = position - position_des;
dot_err_p = linear_vel - vel_linear_des;

uT  = -transpose(-Kp*err_p -Kv*dot_err_p -mass*g*e_3 + mass*acc_linear_des) * Rb*e_3;

zb_des = -(-Kp*err_p -Kv*dot_err_p -mass*g*e_3 + mass*acc_linear_des)/norm(-Kp*err_p -Kv*dot_err_p -mass*g*e_3 + mass*acc_linear_des);

== matlab function hierarchical_controll/Inner-loop control/Inner-loop control ==
  data: Rb_des output size=[3,3]; omega_bb_des output size=3; tau output size=3; zb_des input size=3; Rb input size=[3,3]; dot_Rb_des input size=[3,3]; omega_bb input size=3; dot_omega_bb_des input size=3; xb_des input size=3; Ib parameter size=[3,3]; err_R output size=3; err_W output size=3; Kr parameter; Kw parameter
function [Rb_des,omega_bb_des,tau,err_R,err_W] = fcn(zb_des,Rb,dot_Rb_des,omega_bb,dot_omega_bb_des,xb_des,Ib, Kr, Kw)

%% WRITE HERE THE INNER-LOOP CONTROL
% zb_des: desired z-axis of the body frame
% Rb: current rotation matrix
% dot_Rb_des: time-derivative of the desired rotation matrix
% omega_bb: current angular velocity expressed in the body frame
% dot_omega_bb_des: desired angular acceleration expressed in the body
% frame
% xb_des: desired x-axis of the body frame form the planner
% Ib: inertia matrix of the UAV with respect to the body frame
% ---
% Rb_des: desired rotation matrix
% omega_bb_des: desired angular velocity expressed in the body frame (given
% below as a hint)
% tau: commanded control torque
% err_R: rotational error in SO(3)
% err_W: angular velocity error in SO(3)

yb_des = (skew(zb_des)*xb_des)/norm(skew(zb_des)*xb_des);

Rb_des = [skew(yb_des)*zb_des yb_des zb_des];
omega_bb_des = wedge(Rb_des'*dot_Rb_des);

err_R = wedge(transpose(Rb_des)*Rb - transpose(Rb)*Rb_des);
err_W = omega_bb - transpose(Rb)*Rb_des*omega_bb_des;

tau = -Kr*err_R - Kw*err_W + skew(omega_bb)*Ib*omega_bb - Ib*(skew(omega_bb)*transpose(Rb)*Rb_des*omega_bb_des - transpose(Rb)*Rb_des*dot_omega_bb_des);


end

function S = skew(v)
if(numel(v)~= 1)
S= [0 -v(3) v(2); 
    v(3) 0 -v(1);
    -v(2) v(1) 0];
else
S= zeros(3);
end
end

function v = wedge(S)
v1 = S(3,2);
v2 = S(1,3);
v3 = S(2,1);
v = [v1 v2 v3]';
end

== matlab function hierarchical_controll/Quadrotor dynamics/MATLAB Function1 ==
  data: Rb_temp input; Rb output
function Rb = fcn(Rb_temp)
    [U,S,V] = svd(Rb_temp);
    sigma = det(U*V');
    S_ = diag([1 1 sigma]);

    Rb = U*S_*V';
end

== matlab function hierarchical_controll/1                                                               /MATLAB Function ==
  data: ep input; ud output; edotp input; ad input; newKP parameter
function ud = fcn(ep,edotp,ad, newKP)

new_e=[ep; edotp];


ud = -newKP*new_e+ad;
